simulink model "PID_Classical"  (R2024a)
settings: Solver=VariableStepAuto  StartTime=0.0  StopTime=20  RelTol=1e-3
settings Model: Creator=erhan  LastModifiedBy=erhan

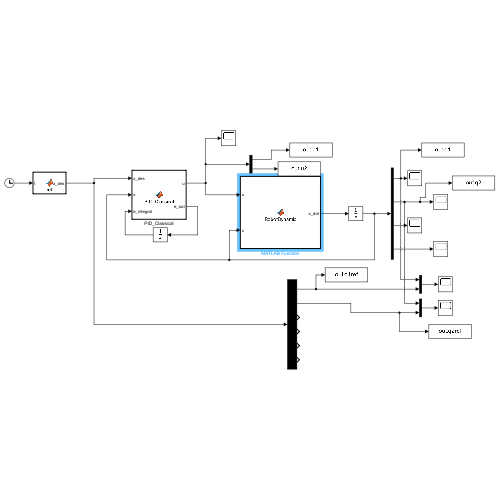
[thumbnail: Simulink's stored preview of the top-level diagram]
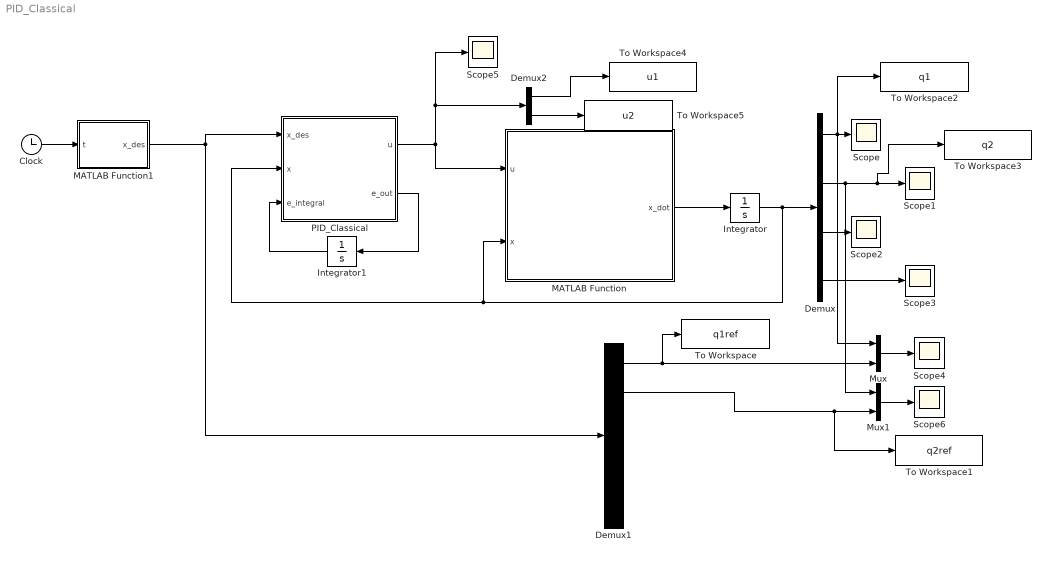
== system PID_Classical ==
  Clock : Clock
  Demux : Demux
  Demux1 : Demux  Outputs=6
  Demux2 : Demux  Outputs=2
  Integrator : Integrator  InitialCondition=[0;0;0;0]
  Integrator1 : Integrator  InitialCondition=[0;0]
  MATLAB Function : MATLAB Function  TreatAsAtomicUnit=on
  MATLAB Function1 : MATLAB Function  TreatAsAtomicUnit=on
  Mux : Mux  Inputs=2
  Mux1 : Mux  Inputs=2
  PID_Classical : MATLAB Function  TreatAsAtomicUnit=on
  Scope{,1..6} (7 alike) : Scope
  To Workspace : ToWorkspace  VariableName=q1ref  SaveFormat=Timeseries  SampleTime=-1
  To Workspace1 : ToWorkspace  VariableName=q2ref  SaveFormat=Timeseries  SampleTime=-1
  To Workspace2 : ToWorkspace  VariableName=q1  SaveFormat=Timeseries  SampleTime=-1
  To Workspace3 : ToWorkspace  VariableName=q2  SaveFormat=Timeseries  SampleTime=-1
  To Workspace4 : ToWorkspace  VariableName=u1  SaveFormat=Timeseries  SampleTime=-1
  To Workspace5 : ToWorkspace  VariableName=u2  SaveFormat=Timeseries  SampleTime=-1
  wires:
  MATLAB Function/1(x_dot) -> Integrator/1
  Integrator/1 -> Demux/1, PID_Classical/2(x), MATLAB Function/2(x)
  Demux/1 -> To Workspace2/1, Mux/1, Scope/1
  Demux/2 -> To Workspace3/1, Scope1/1, Mux1/1
  Demux/3 -> Scope2/1
  Demux/4 -> Scope3/1
  PID_Classical/1(u) -> MATLAB Function/1(u), Demux2/1, Scope5/1
  MATLAB Function1/1(x_des) -> Demux1/1, PID_Classical/1(x_des)
  Clock/1 -> MATLAB Function1/1(t)
  Mux/1 -> Scope4/1
  Demux1/1 -> To Workspace/1, Mux/2
  Demux1/2 -> To Workspace1/1, Mux1/2
  Mux1/1 -> Scope6/1
  PID_Classical/2(e_out) -> Integrator1/1
  Integrator1/1 -> PID_Classical/3(e_integral)
  Demux2/2 -> To Workspace5/1
  Demux2/1 -> To Workspace4/1

== matlab function PID_Classical/PID_Classical ==
  data: x_des input; u output; x input; e_integral input; e_out output
function [u, e_out] = PID_Classical(x_des, x, e_integral)
% GİRİŞLER:
% x_des     : [6x1] (qd1, qd2, dqd1, dqd2, ddqd1, ddqd2)
% x         : [4x1] (q1, q2, dq1, dq2)
% e_integral: [2x1] (Hatanın İntegrali - Simulink Integrator bloğundan gelecek)

% ÇIKIŞLAR:
% u     : [2x1] Torklar
% e_out : [2x1] Anlık Hata (Bunu dışarıda Integrate edeceksiniz)

% --- PARAMETRELER ---


% Kazançlar
Kp = 120;
Kd = 60;
Ki = 30; % İntegral Kazancı

% --- SİNYALLERİ AYRIŞTIRMA ---
qd   = x_des(1:2);   % Hedef Pozisyon
qdp  = x_des(3:4);   % Hedef Hız


q_act  = x(1:2);     % Gerçek Pozisyon
dq_act = x(3:4);     % Gerçek Hız

% --- HATA HESABI ---
e  = qd - q_act;      % Konum Hatası
ep = qdp - dq_act;    % Hız Hatası

% İntegral için dışarıya hata gönderiyoruz
e_out = e; 

s1 =Kd*ep(1) + Kp*e(1) + Ki*e_integral(1);
s2 =Kd*ep(2) + Kp*e(2) + Ki*e_integral(2);

% Tork Hesabı: tau = M*s + N
tau1 = s1;
tau2 = s2;

u = [tau1; tau2];

end

== matlab function PID_Classical/MATLAB Function ==
  data: u input; x_dot output; x input
function x_dot = RobotDynamic(u,x)
% Parametreler
m1=0.8; m2=2.3;
L1=1; L2=1;
g=9.81;

% --- M (Atalet) Matrisi ---
M11 = (L1^2*m1)/3 + L1^2*m2 + (L2^2*m2)/3 + L1*L2*m2*cos(x(2));
M12 = (L2*m2*(2*L2 + 3*L1*cos(x(2))))/6;
M21 = M12;
M22 = (L2^2*m2)/3;

% --- C (Coriolis/Merkezkaç) Vektörü ---
C1 = -(L1*L2*x(3)*m2*sin(x(2))*(2*x(3) + x(4)))/2;
C2 = (L1*L2*x(3)^2*m2*sin(x(2)))/2;

% --- G (Yerçekimi) Vektörü ---
G1 = (g*(L2*m2*cos(x(1) + x(2)) + L1*m1*cos(x(1)) + 2*L1*m2*cos(x(1))))/2;
G2 = (L2*g*m2*cos(x(1) + x(2)))/2;


% N (Nonlinear Terms)
N1 = G1 + C1;
N2 = G2 + C2;

% --- MATRİS TERSİ (Inverse Matrix) HESABI ---
% Determinant
det = M11*M22 - M12*M21;

% HATA BURADAYDI (Düzeltildi)
MI11 = M22/det;
MI12 = -M12/det;
MI21 = -M21/det;  % Eksikti, eklendi.
MI22 = M11/det;   % MI11 yerine MI22 yazildi.

% Giriş Torkları
tau1 = u(1);
tau2 = u(2);

% --- İVMELERİN HESAPLANMASI ---
% Denklem: ddq = inv(M) * (tau - N)
% q(3) -> ddq1
% q(4) -> ddq2

q = zeros(4,1);
q(1) = x(3); % dq1
q(2) = x(4); % dq2

% Matris çarpımı (Manuel):
% ddq1 = MI11*(tau1 - N1) + MI12*(tau2 - N2)
q(3) = MI11*(tau1 - N1) + MI12*(tau2 - N2);

% ddq2 = MI21*(tau1 - N1) + MI22*(tau2 - N2)
q(4) = MI21*(tau1 - N1) + MI22*(tau2 - N2);

x_dot = q;
end

== matlab function PID_Classical/MATLAB Function1 ==
  data: t input; x_des output
function x_des = ref(t)


period = 2;
% amp1 = 0.1;
% amp2 = 0.1;
fact = 2*pi/period;
% sinf = sin(fact*t);
% cosf = cos(fact*t);
qd = [1 1];
qdp = fact*[0 0];
qdpp = -fact^2*qd;
x_des = [qd qdp qdpp]';




end
